simulink model "Sync_machine_blank_model_v1"  (R2021a)
settings: Solver=VariableStepAuto  StartTime=0.0  StopTime=inf  FixedStep=1e-5  MaxStep=100e-6  RelTol=1e-3
libraries: spsGroundLib x5, simulink x3, spsVoltageMeasurementLib x3, spsDCVoltageSourceLib x2, spsThreePhaseBreakerLib x2, spsFourierLib x2, spsThreePhaseVIMeasurementLib x2, spsBreakerLib x2, spsDCMachineLib x1, spsThreePhaseSourceLib x1, spsThreePhaseParallelRLCBranchLib x1, spsRMSLib x1
settings Model: NumberOfSteps=10  Creator=sayan  LastModifiedBy=mansi
settings SolverCC: InitialStep=100e-6  ZeroCrossControl=DisableAll  AlgebraicLoopSolver=TrustRegion
settings DataIOCC: SaveFinalState=on  SaveOutput=off  SaveState=on  SignalLogging=off  DSMLogging=off  ReturnWorkspaceOutputs=off
settings DebuggingCC: MaxConsecutiveZCsMsg=warning  ModelReferenceExtraNoncontSigs=warning  SFMachineParentedDataDiag=warning  ArithmeticOperatorsInVariantConditions=warning
settings SFSimCC: CustomCodeUndefinedFunction=UseInterfaceOnly

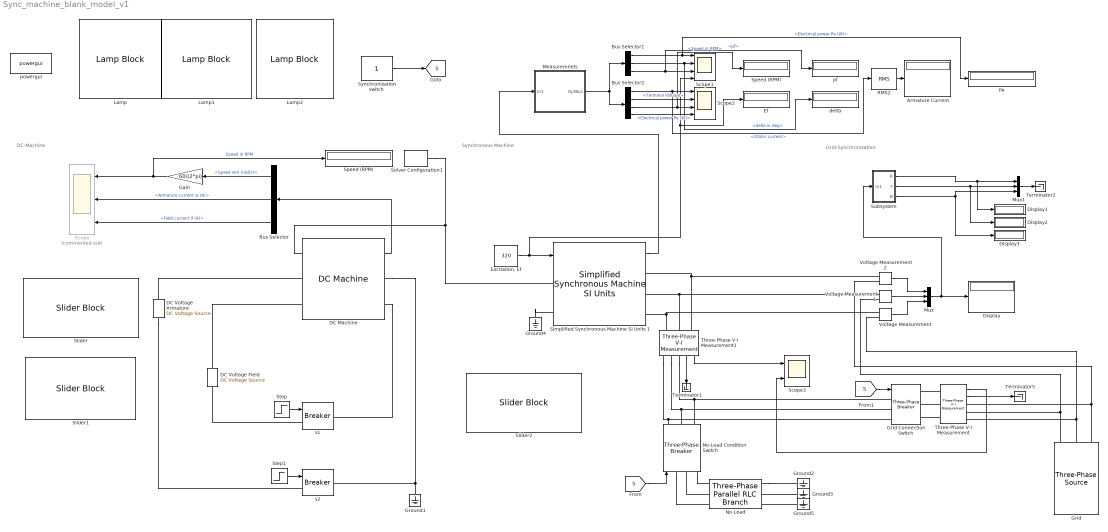
== system Sync_machine_blank_model_v1 ==
  note: Grid-Synchronization
  note: Synchronous Machine
  note: DC-Machine
  Armature Current : Display
  Bus Selector : BusSelector  OutputSignals=Speed wm (rad/s),Armature current ia (A),Field current if (A)
  Bus Selector1 : BusSelector  OutputSignals=signal1.Electrical power Pe (W),signal1.delta in deg,signal1.pf
  Bus Selector2 : BusSelector  OutputSignals=signal2.Stator current,signal2.Terminal Voltage,signal2.Speed in RPM,signal2.Electrical power Pe (W)
  "DC Machine " : spsDCMachineLib/DC Machine  PresetModel=No  MechanicalLoad=Mechanical rotational port  FieldType=Wound  ShowDetailedParameters=on  MeasurementBus=off  RLa=[0.4114*2 0.004895]  RLf=[105.9/2 27.65]  Laf=0.4038  MachineConstant=Torque constant (N.m/A)  Ke=1.8  Kt=1.8  J=0.08321  Bm=0.004313  Tf=2.105  w0=1  Ifinit=1  TsPowergui=0  TsBlock=-1
  DC Voltage Armature : spsDCVoltageSourceLib/DC Voltage Source  Amplitude=300  Measurements=None
  "DC Voltage Field " : spsDCVoltageSourceLib/DC Voltage Source  Amplitude=280.6  Measurements=None
  Display{,1..3} (4 alike) : Display
  Ef : Display
  "Excitation, Ef" : Constant  Value=320
  Gain : Gain  Gain=60/(2*pi)
  Grid : spsThreePhaseSourceLib/Three-Phase Source  InternalConnection=Yg  VoltagePhases=off  Voltage=400  PhaseAngle=0  Voltage_phases=[25e3 25e3 25e3]/sqrt(3)  PhaseAngles_phases=[0 -120 +120]  Frequency=50  NonIdealSource=on  SpecifyImpedance=off  Resistance=0.08929  Inductance=16.58e-3  ShortCircuitLevel=100e6  BaseVoltage=400  XRratio=7  BusType=swing  Pref=10e3  Qref=0  Prefabc=[10e3, 10e3, 10e3]  Qrefabc=[0, 0, 0]  Qmin=-inf  Qmax=inf
  Grid Connection Switch : spsThreePhaseBreakerLib/Three-Phase Breaker  InitialState=open  SwitchA=on  SwitchB=on  SwitchC=on  SwitchTimes="[1/60  5/60]"  External=on  BreakerResistance=0  SnubberResistance=1e8  SnubberCapacitance=inf  Measurements=None
  Ground{1..5} (5 alike) : spsGroundLib/Ground  LConnTagsString=a
  Lamp : LampBlock
  Lamp1 : LampBlock
  Lamp2 : LampBlock
  Measuremnets : Subsystem
  Mux : Mux  Inputs=3
  Mux1 : Mux  Inputs=3
  No-Load : spsThreePhaseParallelRLCBranchLib/Three-Phase Parallel RLC Branch  LConnTagsString=A|B|C  RConnTagsString=A|B|C  BranchType=R  Resistance=1e6  Inductance=1e-3  Capacitance=1e-6  Measurements=None
      settings: SourceProductBaseCode=PS
  No-Load Condition Switch : spsThreePhaseBreakerLib/Three-Phase Breaker  InitialState=closed  SwitchA=on  SwitchB=on  SwitchC=on  SwitchTimes="[1/60  5/60]"  External=on  BreakerResistance=0  SnubberResistance=1e8  SnubberCapacitance=inf  Measurements=None
  Pe : Display
  RMS2 : spsRMSLib/RMS  TrueRMS=off  Freq=50  RMSInit=0  Ts=0
  Scope : Scope  Commented=on  NumInputPorts=3
  Scope1 : Scope  NumInputPorts=4
  Scope2 : Scope  NumInputPorts=4
  Scope3 : Scope  NumInputPorts=2
  Simplified Synchronous Machine SI Units 1 : spsSimplifiedSynchronousMachineSIUnitsLib/Simplified Synchronous Machine SI Units  ConnectionType=4-wire Y  MechanicalLoad=Mechanical rotational port  MeasurementBus=off  NominalParameters=[20e3 400 50]  Mechanical=[0.124 0 2]  InternalRL="[0.204  0.8104e-3]"  InitialConditions="[ 0,0   0,0,0   0,0,0 ]"  IterativeDiscreteModel=Trapezoidal non iterative  TsBlock=-1  TsPowergui=0  LoadFlowParameters=[1,0,0,0,0]  Units=1  BusType=swing  Pref=0  Qref=0  Qmin=-inf  Qmax=+inf  PLF=0  QLF=0
      settings: SourceProductBaseCode=PS
  Slider : SliderBlock  ScaleMax=300
  Slider1 : SliderBlock  ScaleMax=300
  Slider2 : SliderBlock  ScaleMax=600
  Solver Configuration1 : nesl_utility/Solver Configuration  PhysicalDomain=network_engine_domain  SubClassName=solver  LeftPortType=input  RightPortType=generic  Tones=[]  Harmonics=[]  SimulateNoise=off  Profile=off  UseLocalSampling=off  EnableSwitchedLinearOptims=on  FrequencyDomain=off  UseCCode=off  RelTol=0.001  AbsTol=1e-06  MinStep=1e-09  ToWorkspace=off  RevertToSquareIcSolve=off  NumHomotopyIterations=100  PhasorMode=off  PhasorModeNumHarmonics=1  DoDC=off  ResidualTolerance=1e-09  UseLocalSolver=off  LocalSolverChoice=NE_BACKWARD_EULER_ADVANCER  LocalSolverSampleTime=0.001  DoFixedCost=off  MaxNonlinIter=3  MaxModeIter=2  ComputeImpulses=off  ImpulseIterations=2  LinearAlgebra=Sparse  EquationFormulation=NE_TIME_EF  DelaysMemoryBudget=1024  AutomaticFiltering=on  FilteringTimeConstant=0.001  PartitionStorageMethod=AS_NEEDED  PartitionMemoryBudget=1024  PartitionMethod=FAST
      settings: SourceProductBaseCode=PW,SS
  Speed (RPM) : Display
  "Speed (RPM) " : Display
  Step : Step  Time=0  SampleTime=0
  Step1 : Step  Time=0.0001  SampleTime=0
  Subsystem : Subsystem
  Synchronization switch : Constant
  Terminator1 : Terminator
  Terminator2 : Terminator
  Terminator5 : Terminator
  Three-Phase V-I Measurement : spsThreePhaseVIMeasurementLib/Three-Phase V-I Measurement  VoltageMeasurement=phase-to-phase  SetLabelV=off  LabelV=Vabc  Vpu=off  VpuLL=off  CurrentMeasurement=yes  SetLabelI=off  LabelI=Iabc  Ipu=off  Pbase=100e6  Vbase=500e3  OutputType=Complex  PhasorSimulation=off  PSBequivalent=0
  Three-Phase V-I Measurement1 : spsThreePhaseVIMeasurementLib/Three-Phase V-I Measurement  VoltageMeasurement=phase-to-phase  SetLabelV=off  LabelV=Vabc  Vpu=off  VpuLL=off  CurrentMeasurement=yes  SetLabelI=off  LabelI=Iabc  Ipu=off  Pbase=100e6  Vbase=500e3  OutputType=Complex  PhasorSimulation=off  PSBequivalent=0
  Voltage Measurement : spsVoltageMeasurementLib/Voltage Measurement  PhasorSimulation=off  OutputType=Complex  PSBequivalent=0
  Voltage Measurement1 : spsVoltageMeasurementLib/Voltage Measurement  PhasorSimulation=off  OutputType=Complex  PSBequivalent=0
  Voltage Measurement2 : spsVoltageMeasurementLib/Voltage Measurement  PhasorSimulation=off  OutputType=Complex  PSBequivalent=0
  delta : Display
  pf : Display
  powergui : spspowerguiLib/powergui  Priority=1  SimulationMode=Continuous  SampleTime=1e-5  frequency=60  Iterations=50  frequencyindice=0  Pbase=100e6  ErrMax=1e-4  UnitsV=kV  UnitsW=MW  buscounter=0  FunctionMessages=off  echomessages=off  EnableUseOfTLC=off  CurrentSourceSwitches=off  DisableSnubberDevices=off  DisableRonSwitches=off  DisableVfSwitches=off  DisplayEquations=off  AutomaticDiscreteSolvers=off  SolverType=Tustin/Backward Euler (TBE)  Interpol=off  ExternalGateDelay=off  methode=off  Ts=100  x0status=blocks  SPID=off  SwTol=0  HookPort=off  NonlinearTolerance=1e-4  nMaxIteration=100  ContinueOnMaxIteration=off  RestoreLinks=warning  ResistiveCurrentMeasurement=off  Frange=[0:2:500]  Ylog=off  Xlog=on  ShowGrid=off  save=off  variable=ZData  structure=0  ZoomFFT=off  StartTime=0.0  cycles=1  DisplayStyle=1  fundamental=60  FreqAxis=off  MaxFrequency=1000  frequencyindicesteady=1  RmsSteady=1  display=off
  s1 : spsBreakerLib/Breaker  InitialState=0  SwitchingTimes="[1/60  5/60]"  External=on  BreakerResistance=0.01  SnubberResistance=inf  SnubberCapacitance=inf  Measurements=None  MoreParameters=on  NoBreakLoop=off
      settings: SourceProductBaseCode=PS
  s2 : spsBreakerLib/Breaker  InitialState=0  SwitchingTimes="[1/60  5/60]"  External=on  BreakerResistance=0.01  SnubberResistance=inf  SnubberCapacitance=inf  Measurements=None  MoreParameters=on  NoBreakLoop=off
      settings: SourceProductBaseCode=PS
  tag scope: S=global
  wires:
  "DC Machine "/1 -> Bus Selector/1
  Bus Selector/1 -> Gain/1  "<Speed wm (rad/s)>"
  Bus Selector/2 -> Scope/2  "<Armature current ia (A)>"
  Gain/1 -> "Speed (RPM) "/1, Scope/1  "Speed in RPM"
  Bus Selector/3 -> Scope/3  "<Field current if (A)>"
  Step/1 -> s1/1
  Step1/1 -> s2/1
  Three-Phase V-I Measurement/1 -> Scope3/2
  Simplified Synchronous Machine SI Units 1/1 -> Measuremnets/1(In1)
  Measuremnets/1(OutBus) -> Bus Selector1/1, Bus Selector2/1
  Bus Selector1/1 -> Scope1/1, Pe/1  "<Electrical power Pe (W)>"
  Bus Selector1/2 -> delta/1, Scope1/2  "<delta in deg>"
  Bus Selector1/3 -> pf/1, Scope1/3  "<pf>"
  Bus Selector2/1 -> RMS2/1, Scope2/1  "<Stator current>"
  Bus Selector2/2 -> Scope2/2  "<Terminal Voltage>"
  Bus Selector2/3 -> Scope2/3, Speed (RPM)/1  "<Speed in RPM>"
  Bus Selector2/4 -> Scope2/4  "<Electrical power Pe (W)>"
  Three-Phase V-I Measurement/2 -> Terminator5/1
  RMS2/1 -> Armature Current/1
  "Excitation, Ef"/1 -> Scope1/4, Ef/1, Simplified Synchronous Machine SI Units 1/1
  Synchronization switch/1 -> [S]
  [S] -> No-Load Condition Switch/1
  [S] -> Grid Connection Switch/1
  Three-Phase V-I Measurement1/1 -> Scope3/1
  Three-Phase V-I Measurement1/2 -> Terminator1/1
  Voltage Measurement2/1 -> Mux/1
  Voltage Measurement1/1 -> Mux/2
  Voltage Measurement/1 -> Mux/3
  Mux/1 -> Subsystem/1(In1), Display/1
  Mux1/1 -> Terminator2/1
  Subsystem/1(R) -> Display1/1, Mux1/1
  Subsystem/2(Y) -> Display2/1, Mux1/2
  Subsystem/3(B) -> Display3/1, Mux1/3
  connections:
  "DC Machine "/RConn1 -- Ground1/LConn1 -- s2/RConn1
  Solver Configuration1/RConn1 -- Simplified Synchronous Machine SI Units 1/LConn1 -- "DC Machine "/LConn1
  "DC Machine "/RConn2 -- s1/RConn1
  Grid/RConn3 -- Voltage Measurement2/LConn2 -- Three-Phase V-I Measurement/RConn1
  Grid Connection Switch/LConn3 -- Three-Phase V-I Measurement1/RConn3 -- No-Load Condition Switch/RConn1
  Three-Phase V-I Measurement/LConn1 -- Grid Connection Switch/RConn1
  Three-Phase V-I Measurement/LConn2 -- Grid Connection Switch/RConn2
  Three-Phase V-I Measurement/LConn3 -- Grid Connection Switch/RConn3
  No-Load/LConn2 -- No-Load Condition Switch/LConn2
  Ground4/LConn1 -- Simplified Synchronous Machine SI Units 1/LConn2
  No-Load/RConn1 -- Ground2/LConn1
  Ground3/LConn1 -- No-Load/RConn2
  Ground5/LConn1 -- No-Load/RConn3
  Grid/RConn1 -- Voltage Measurement1/LConn2 -- Three-Phase V-I Measurement/RConn2
  Grid/RConn2 -- Voltage Measurement/LConn2 -- Three-Phase V-I Measurement/RConn3
  No-Load Condition Switch/LConn3 -- No-Load/LConn1
  No-Load Condition Switch/LConn1 -- No-Load/LConn3
  DC Voltage Armature/RConn1 -- "DC Machine "/LConn2
  DC Voltage Armature/LConn1 -- s2/LConn1
  "DC Voltage Field "/RConn1 -- "DC Machine "/LConn3
  s1/LConn1 -- "DC Voltage Field "/LConn1
  Grid Connection Switch/LConn2 -- Three-Phase V-I Measurement1/RConn2 -- No-Load Condition Switch/RConn2
  Grid Connection Switch/LConn1 -- No-Load Condition Switch/RConn3 -- Three-Phase V-I Measurement1/RConn1
  Three-Phase V-I Measurement1/LConn2 -- Voltage Measurement1/LConn1 -- Simplified Synchronous Machine SI Units 1/RConn2
  Three-Phase V-I Measurement1/LConn3 -- Voltage Measurement/LConn1 -- Simplified Synchronous Machine SI Units 1/RConn3
  Three-Phase V-I Measurement1/LConn1 -- Voltage Measurement2/LConn1 -- Simplified Synchronous Machine SI Units 1/RConn1

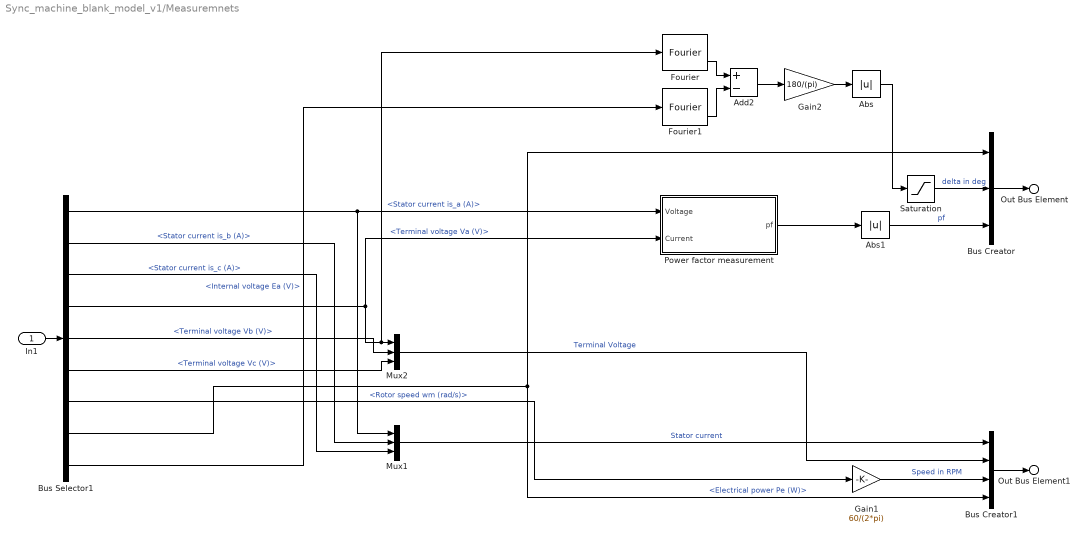
== system Sync_machine_blank_model_v1/Measuremnets ==
  In1 : Inport
  Abs : Abs
  Abs1 : Abs
  Add2 : Sum  Inputs=+-
  Bus Creator : BusCreator  Inputs=3
  Bus Creator1 : BusCreator  Inputs=4
  Bus Selector1 : BusSelector  OutputSignals=Stator current is_a (A),Stator current is_b (A),Stator current is_c (A),Terminal voltage Va (V),Terminal voltage Vb (V),Terminal voltage Vc (V),Rotor speed wm (rad/s),Electrical power Pe (W),Internal voltage Ea (V)
  Fourier : spsFourierLib/Fourier  Freq=50  n=1  InInit=[0, 0]  Ts=0
      settings: SourceProductBaseCode=PS
  Fourier1 : spsFourierLib/Fourier  Freq=50  n=1  InInit=[0, 0]  Ts=0
      settings: SourceProductBaseCode=PS
  Gain1 : Gain  Gain=60/(2*pi)
  Gain2 : Gain  Gain=180/(pi)
  Mux1 : Mux  Inputs=3
  Mux2 : Mux  Inputs=3
  Power factor measurement : Subsystem
  Saturation : Saturate  UpperLimit=100  LowerLimit=-100
  Out Bus Element : Outport  VectorParamsAs1DForOutWhenUnconnected=off  PortName=OutBus  Element=signal1
  Out Bus Element1 : Outport  VectorParamsAs1DForOutWhenUnconnected=off  PortName=OutBus  Element=signal2
  wires:
  Bus Selector1/4 -> Fourier/1, Mux2/1, Power factor measurement/2(Current)  "<Terminal voltage Va (V)>"
  Bus Selector1/2 -> Mux1/2  "<Stator current is_b (A)>"
  Bus Selector1/5 -> Mux2/2  "<Terminal voltage Vb (V)>"
  Bus Selector1/8 -> Bus Creator1/4, Bus Creator/1  "<Electrical power Pe (W)>"
  Gain1/1 -> Bus Creator1/3  "Speed in RPM"
  In1/1 -> Bus Selector1/1
  Bus Selector1/9 -> Fourier1/1  "<Internal voltage Ea (V)>"
  Mux1/1 -> Bus Creator1/1  "Stator current"
  Fourier/2 -> Add2/1
  Bus Selector1/1 -> Mux1/1, Power factor measurement/1(Voltage)  "<Stator current is_a (A)>"
  Add2/1 -> Gain2/1
  Bus Selector1/3 -> Mux1/3  "<Stator current is_c (A)>"
  Bus Selector1/6 -> Mux2/3  "<Terminal voltage Vc (V)>"
  Mux2/1 -> Bus Creator1/2  "Terminal Voltage"
  Bus Selector1/7 -> Gain1/1  "<Rotor speed wm (rad/s)>"
  Fourier1/2 -> Add2/2
  Gain2/1 -> Abs/1
  Bus Creator/1 -> Out Bus Element/1
  Bus Creator1/1 -> Out Bus Element1/1
  Saturation/1 -> Bus Creator/2  "delta in deg"
  Power factor measurement/1(pf) -> Abs1/1
  Abs/1 -> Saturation/1
  Abs1/1 -> Bus Creator/3  "pf"

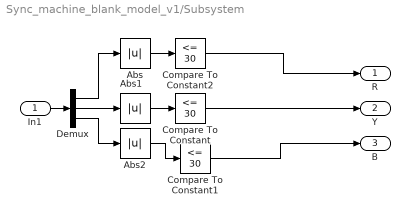
== system Sync_machine_blank_model_v1/Subsystem ==
  In1 : Inport
  Abs : Abs
  Abs1 : Abs
  Abs2 : Abs
  Compare To Constant : simulink/Logic and Bit Operations/Compare To Constant  relop=<=  const=30  OutDataTypeStr=boolean
  Compare To Constant1 : simulink/Logic and Bit Operations/Compare To Constant  relop=<=  const=30  OutDataTypeStr=boolean
  Compare To Constant2 : simulink/Logic and Bit Operations/Compare To Constant  relop=<=  const=30  OutDataTypeStr=boolean
  Demux : Demux  Outputs=3
  R : Outport
  Y : Outport  Port=2
  B : Outport  Port=3
  wires:
  In1/1 -> Demux/1
  Demux/1 -> Abs/1
  Demux/2 -> Abs1/1
  Demux/3 -> Abs2/1
  Abs2/1 -> Compare To Constant1/1
  Abs1/1 -> Compare To Constant/1
  Abs/1 -> Compare To Constant2/1
  Compare To Constant1/1 -> B/1
  Compare To Constant/1 -> Y/1
  Compare To Constant2/1 -> R/1

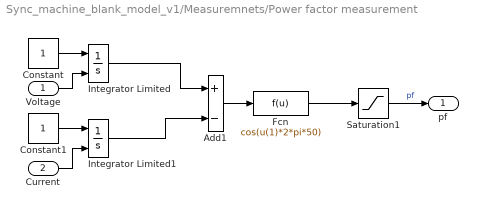
== system Sync_machine_blank_model_v1/Measuremnets/Power factor measurement ==
  Voltage : Inport
  Current : Inport  Port=2
  Add1 : Sum  Inputs=+-
  Constant : Constant
  Constant1 : Constant
  Fcn : Fcn  Expr=cos(u(1)*2*pi*50)
  Integrator Limited : Integrator  ExternalReset=falling  UpperSaturationLimit=1  LowerSaturationLimit=0
  Integrator Limited1 : Integrator  ExternalReset=falling  UpperSaturationLimit=1  LowerSaturationLimit=0
  Saturation1 : Saturate  UpperLimit=1.5  LowerLimit=-1.5
  pf : Outport  VectorParamsAs1DForOutWhenUnconnected=off
  wires:
  Add1/1 -> Fcn/1
  Constant/1 -> Integrator Limited/1
  Integrator Limited1/1 -> Add1/2
  Fcn/1 -> Saturation1/1
  Saturation1/1 -> pf/1  "pf"
  Integrator Limited/1 -> Add1/1
  Voltage/1 -> Integrator Limited/2
  Constant1/1 -> Integrator Limited1/1
  Current/1 -> Integrator Limited1/2
